simulink library "batt_packBTMSExampleLib"  (R2023a)
settings: Solver=VariableStepAuto  StartTime=0.0  StopTime=10.0  RelTol=1e-3
libraries: batt_packBTMSExampleLib_lib x12
(part 2 of 2)

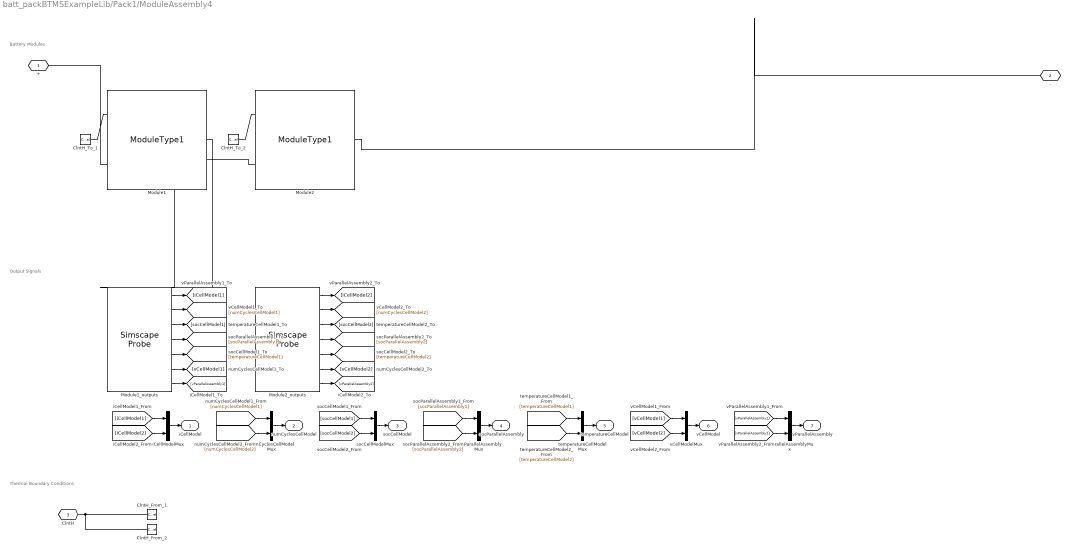
== system batt_packBTMSExampleLib/Pack1/ModuleAssembly4 ==
  note: Thermal Boundary Conditions
  note: Output Signals
  note: Battery Modules
  ClntH_From_1 : ConnectionLabel  Label=clntH_1
  ClntH_From_2 : ConnectionLabel  Label=clntH_2
  ClntH_To_1 : ConnectionLabel  Label=clntH_1
  ClntH_To_2 : ConnectionLabel  Label=clntH_2
  Module1 : batt_packBTMSExampleLib_lib/Modules/ModuleType1  SOC_vec=ModuleType1.SOC_vec  T_vec=ModuleType1.T_vec K  V0_mat=ModuleType1.V0_mat V  V_range=ModuleType1.V_range V  R0_mat=ModuleType1.R0_mat Ohm  AH=ModuleType1.AH A*hr  extrapolation_option=simscape.enum.extrapolation.nearest  thermal_mass=ModuleType1.thermal_mass J/K  CoolantThermalPathResistance=ModuleType1.CoolantThermalPathResistance K/W  P=3  S=11  iCellModel_specify=on  iCellModel_priority=None  iCellModel=ModuleAssembly4.Module1.iCellModel A  iCellModel_nominal_specify=off  iCellModel_nominal_unit=A  iCellModel_nominal_value=1  vCellModel_specify=on  vCellModel_priority=None  vCellModel=ModuleAssembly4.Module1.vCellModel V  vCellModel_nominal_specify=off  vCellModel_nominal_unit=V  vCellModel_nominal_value=1  socCellModel_specify=on  socCellModel_priority=High  socCellModel=ModuleAssembly4.Module1.socCellModel  socCellModel_nominal_specify=off  socCellModel_nominal_unit=1  socCellModel_nominal_value=1  numCyclesCellModel_specify=on  numCyclesCellModel_priority=High  numCyclesCellModel=ModuleAssembly4.Module1.numCyclesCellModel  numCyclesCellModel_nominal_specify=off  numCyclesCellModel_nominal_unit=1  numCyclesCellModel_nominal_value=1  temperatureCellModel_specify=on  temperatureCellModel_priority=High  temperatureCellModel=ModuleAssembly4.Module1.temperatureCellModel K  temperatureCellModel_nominal_specify=off  temperatureCellModel_nominal_unit=K  temperatureCellModel_nominal_value=1  vParallelAssembly_specify=on  vParallelAssembly_priority=None  vParallelAssembly=ModuleAssembly4.Module1.vParallelAssembly V  vParallelAssembly_nominal_specify=off  vParallelAssembly_nominal_unit=V  vParallelAssembly_nominal_value=1  socParallelAssembly_specify=on  socParallelAssembly_priority=None  socParallelAssembly=ModuleAssembly4.Module1.socParallelAssembly  socParallelAssembly_nominal_specify=off  socParallelAssembly_nominal_unit=1  socParallelAssembly_nominal_value=1
      settings: InternalSimscapePortConfiguration="{\"Bottom\":[{\"id\":\"n\",\"label\":\"-\",\"type\":\"foundation.electrical.electrical\"}],\"Left\":[{\"id\":\"ClntH\",\"label\":\"CH\",\"type\":\"foundation.thermal.thermal\"}],\"Right\":[],\"Top\":[{\"id\":\"p\",\"label\":\"+\",\"type\":\"foundation.electrical.electrical\"}]}"
  Module1_outputs : SimscapeProbe  BoundBlock=236  Variables={iCellModel, numCyclesCellModel, socCellModel, socParallelAssembly, temperatureCellModel, vCellModel, vParallelAssembly}
  Module2 : batt_packBTMSExampleLib_lib/Modules/ModuleType1  SOC_vec=ModuleType1.SOC_vec  T_vec=ModuleType1.T_vec K  V0_mat=ModuleType1.V0_mat V  V_range=ModuleType1.V_range V  R0_mat=ModuleType1.R0_mat Ohm  AH=ModuleType1.AH A*hr  extrapolation_option=simscape.enum.extrapolation.nearest  thermal_mass=ModuleType1.thermal_mass J/K  CoolantThermalPathResistance=ModuleType1.CoolantThermalPathResistance K/W  P=3  S=11  iCellModel_specify=on  iCellModel_priority=None  iCellModel=ModuleAssembly4.Module2.iCellModel A  iCellModel_nominal_specify=off  iCellModel_nominal_unit=A  iCellModel_nominal_value=1  vCellModel_specify=on  vCellModel_priority=None  vCellModel=ModuleAssembly4.Module2.vCellModel V  vCellModel_nominal_specify=off  vCellModel_nominal_unit=V  vCellModel_nominal_value=1  socCellModel_specify=on  socCellModel_priority=High  socCellModel=ModuleAssembly4.Module2.socCellModel  socCellModel_nominal_specify=off  socCellModel_nominal_unit=1  socCellModel_nominal_value=1  numCyclesCellModel_specify=on  numCyclesCellModel_priority=High  numCyclesCellModel=ModuleAssembly4.Module2.numCyclesCellModel  numCyclesCellModel_nominal_specify=off  numCyclesCellModel_nominal_unit=1  numCyclesCellModel_nominal_value=1  temperatureCellModel_specify=on  temperatureCellModel_priority=High  temperatureCellModel=ModuleAssembly4.Module2.temperatureCellModel K  temperatureCellModel_nominal_specify=off  temperatureCellModel_nominal_unit=K  temperatureCellModel_nominal_value=1  vParallelAssembly_specify=on  vParallelAssembly_priority=None  vParallelAssembly=ModuleAssembly4.Module2.vParallelAssembly V  vParallelAssembly_nominal_specify=off  vParallelAssembly_nominal_unit=V  vParallelAssembly_nominal_value=1  socParallelAssembly_specify=on  socParallelAssembly_priority=None  socParallelAssembly=ModuleAssembly4.Module2.socParallelAssembly  socParallelAssembly_nominal_specify=off  socParallelAssembly_nominal_unit=1  socParallelAssembly_nominal_value=1
      settings: InternalSimscapePortConfiguration="{\"Bottom\":[{\"id\":\"n\",\"label\":\"-\",\"type\":\"foundation.electrical.electrical\"}],\"Left\":[{\"id\":\"ClntH\",\"label\":\"CH\",\"type\":\"foundation.thermal.thermal\"}],\"Right\":[],\"Top\":[{\"id\":\"p\",\"label\":\"+\",\"type\":\"foundation.electrical.electrical\"}]}"
  Module2_outputs : SimscapeProbe  BoundBlock=238  Variables={iCellModel, numCyclesCellModel, socCellModel, socParallelAssembly, temperatureCellModel, vCellModel, vParallelAssembly}
  iCellModelMux : Mux  Inputs=2
  numCyclesCellModelMux : Mux  Inputs=2
  socCellModelMux : Mux  Inputs=2
  socParallelAssemblyMux : Mux  Inputs=2
  temperatureCellModelMux : Mux  Inputs=2
  vCellModelMux : Mux  Inputs=2
  vParallelAssemblyMux : Mux  Inputs=2
  + : PMIOPort  Side=Left
  - : PMIOPort  Port=2  Side=Right
  ClntH : PMIOPort  Port=3  Side=Right
  iCellModel : Outport
  numCyclesCellModel : Outport  Port=2
  socCellModel : Outport  Port=3
  socParallelAssembly : Outport  Port=4
  temperatureCellModel : Outport  Port=5
  vCellModel : Outport  Port=6
  vParallelAssembly : Outport  Port=7
  wires:
  [vParallelAssembly2] -> vParallelAssemblyMux/2
  Module2_outputs/1 -> [iCellModel2]
  [vCellModel2] -> vCellModelMux/2
  Module2_outputs/2 -> [numCyclesCellModel2]
  [temperatureCellModel2] -> temperatureCellModelMux/2
  Module2_outputs/3 -> [socCellModel2]
  [socParallelAssembly2] -> socParallelAssemblyMux/2
  Module2_outputs/4 -> [socParallelAssembly2]
  [socCellModel2] -> socCellModelMux/2
  Module2_outputs/5 -> [temperatureCellModel2]
  [numCyclesCellModel2] -> numCyclesCellModelMux/2
  Module2_outputs/6 -> [vCellModel2]
  [iCellModel2] -> iCellModelMux/2
  Module2_outputs/7 -> [vParallelAssembly2]
  [vParallelAssembly1] -> vParallelAssemblyMux/1
  vParallelAssemblyMux/1 -> vParallelAssembly/1
  Module1_outputs/1 -> [iCellModel1]
  [vCellModel1] -> vCellModelMux/1
  vCellModelMux/1 -> vCellModel/1
  Module1_outputs/2 -> [numCyclesCellModel1]
  [temperatureCellModel1] -> temperatureCellModelMux/1
  temperatureCellModelMux/1 -> temperatureCellModel/1
  Module1_outputs/3 -> [socCellModel1]
  [socParallelAssembly1] -> socParallelAssemblyMux/1
  socParallelAssemblyMux/1 -> socParallelAssembly/1
  Module1_outputs/4 -> [socParallelAssembly1]
  [socCellModel1] -> socCellModelMux/1
  socCellModelMux/1 -> socCellModel/1
  Module1_outputs/5 -> [temperatureCellModel1]
  [numCyclesCellModel1] -> numCyclesCellModelMux/1
  numCyclesCellModelMux/1 -> numCyclesCellModel/1
  Module1_outputs/6 -> [vCellModel1]
  [iCellModel1] -> iCellModelMux/1
  iCellModelMux/1 -> iCellModel/1
  Module1_outputs/7 -> [vParallelAssembly1]
  connections:
  ClntH_To_2/LConn1 -- Module2/LConn1
  ClntH_From_2/LConn1 -- ClntH_From_1/LConn1 -- ClntH/RConn1
  ClntH_To_1/LConn1 -- Module1/LConn1
  Module2/RConn1 -- -/RConn1
  Module1/LConn2 -- +/RConn1
  Module2/LConn2 -- Module1/RConn1

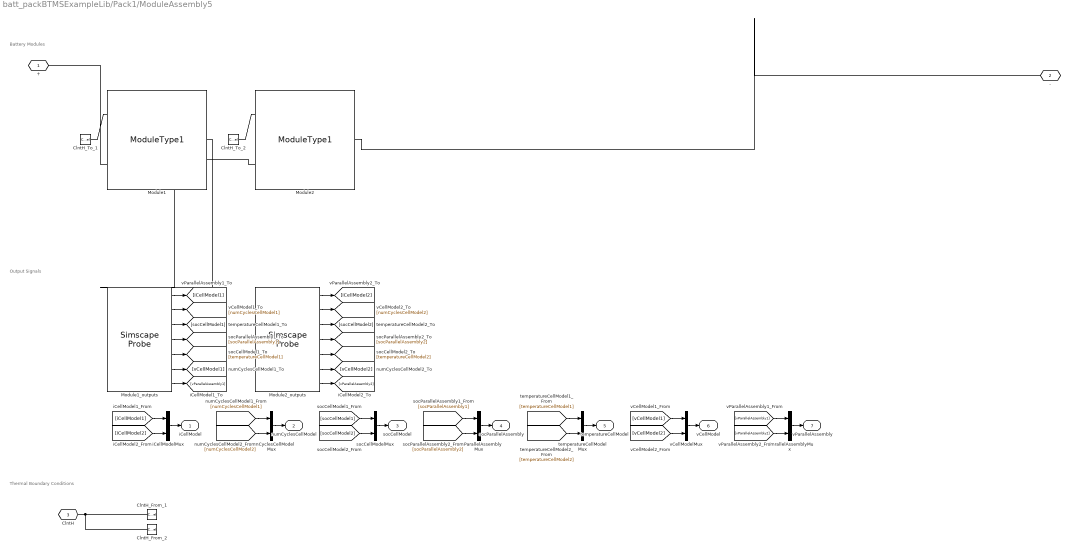
== system batt_packBTMSExampleLib/Pack1/ModuleAssembly5 ==
  note: Thermal Boundary Conditions
  note: Output Signals
  note: Battery Modules
  ClntH_From_1 : ConnectionLabel  Label=clntH_1
  ClntH_From_2 : ConnectionLabel  Label=clntH_2
  ClntH_To_1 : ConnectionLabel  Label=clntH_1
  ClntH_To_2 : ConnectionLabel  Label=clntH_2
  Module1 : batt_packBTMSExampleLib_lib/Modules/ModuleType1  SOC_vec=ModuleType1.SOC_vec  T_vec=ModuleType1.T_vec K  V0_mat=ModuleType1.V0_mat V  V_range=ModuleType1.V_range V  R0_mat=ModuleType1.R0_mat Ohm  AH=ModuleType1.AH A*hr  extrapolation_option=simscape.enum.extrapolation.nearest  thermal_mass=ModuleType1.thermal_mass J/K  CoolantThermalPathResistance=ModuleType1.CoolantThermalPathResistance K/W  P=3  S=11  iCellModel_specify=on  iCellModel_priority=None  iCellModel=ModuleAssembly5.Module1.iCellModel A  iCellModel_nominal_specify=off  iCellModel_nominal_unit=A  iCellModel_nominal_value=1  vCellModel_specify=on  vCellModel_priority=None  vCellModel=ModuleAssembly5.Module1.vCellModel V  vCellModel_nominal_specify=off  vCellModel_nominal_unit=V  vCellModel_nominal_value=1  socCellModel_specify=on  socCellModel_priority=High  socCellModel=ModuleAssembly5.Module1.socCellModel  socCellModel_nominal_specify=off  socCellModel_nominal_unit=1  socCellModel_nominal_value=1  numCyclesCellModel_specify=on  numCyclesCellModel_priority=High  numCyclesCellModel=ModuleAssembly5.Module1.numCyclesCellModel  numCyclesCellModel_nominal_specify=off  numCyclesCellModel_nominal_unit=1  numCyclesCellModel_nominal_value=1  temperatureCellModel_specify=on  temperatureCellModel_priority=High  temperatureCellModel=ModuleAssembly5.Module1.temperatureCellModel K  temperatureCellModel_nominal_specify=off  temperatureCellModel_nominal_unit=K  temperatureCellModel_nominal_value=1  vParallelAssembly_specify=on  vParallelAssembly_priority=None  vParallelAssembly=ModuleAssembly5.Module1.vParallelAssembly V  vParallelAssembly_nominal_specify=off  vParallelAssembly_nominal_unit=V  vParallelAssembly_nominal_value=1  socParallelAssembly_specify=on  socParallelAssembly_priority=None  socParallelAssembly=ModuleAssembly5.Module1.socParallelAssembly  socParallelAssembly_nominal_specify=off  socParallelAssembly_nominal_unit=1  socParallelAssembly_nominal_value=1
      settings: InternalSimscapePortConfiguration="{\"Bottom\":[{\"id\":\"n\",\"label\":\"-\",\"type\":\"foundation.electrical.electrical\"}],\"Left\":[{\"id\":\"ClntH\",\"label\":\"CH\",\"type\":\"foundation.thermal.thermal\"}],\"Right\":[],\"Top\":[{\"id\":\"p\",\"label\":\"+\",\"type\":\"foundation.electrical.electrical\"}]}"
  Module1_outputs : SimscapeProbe  BoundBlock=293  Variables={iCellModel, numCyclesCellModel, socCellModel, socParallelAssembly, temperatureCellModel, vCellModel, vParallelAssembly}
  Module2 : batt_packBTMSExampleLib_lib/Modules/ModuleType1  SOC_vec=ModuleType1.SOC_vec  T_vec=ModuleType1.T_vec K  V0_mat=ModuleType1.V0_mat V  V_range=ModuleType1.V_range V  R0_mat=ModuleType1.R0_mat Ohm  AH=ModuleType1.AH A*hr  extrapolation_option=simscape.enum.extrapolation.nearest  thermal_mass=ModuleType1.thermal_mass J/K  CoolantThermalPathResistance=ModuleType1.CoolantThermalPathResistance K/W  P=3  S=11  iCellModel_specify=on  iCellModel_priority=None  iCellModel=ModuleAssembly5.Module2.iCellModel A  iCellModel_nominal_specify=off  iCellModel_nominal_unit=A  iCellModel_nominal_value=1  vCellModel_specify=on  vCellModel_priority=None  vCellModel=ModuleAssembly5.Module2.vCellModel V  vCellModel_nominal_specify=off  vCellModel_nominal_unit=V  vCellModel_nominal_value=1  socCellModel_specify=on  socCellModel_priority=High  socCellModel=ModuleAssembly5.Module2.socCellModel  socCellModel_nominal_specify=off  socCellModel_nominal_unit=1  socCellModel_nominal_value=1  numCyclesCellModel_specify=on  numCyclesCellModel_priority=High  numCyclesCellModel=ModuleAssembly5.Module2.numCyclesCellModel  numCyclesCellModel_nominal_specify=off  numCyclesCellModel_nominal_unit=1  numCyclesCellModel_nominal_value=1  temperatureCellModel_specify=on  temperatureCellModel_priority=High  temperatureCellModel=ModuleAssembly5.Module2.temperatureCellModel K  temperatureCellModel_nominal_specify=off  temperatureCellModel_nominal_unit=K  temperatureCellModel_nominal_value=1  vParallelAssembly_specify=on  vParallelAssembly_priority=None  vParallelAssembly=ModuleAssembly5.Module2.vParallelAssembly V  vParallelAssembly_nominal_specify=off  vParallelAssembly_nominal_unit=V  vParallelAssembly_nominal_value=1  socParallelAssembly_specify=on  socParallelAssembly_priority=None  socParallelAssembly=ModuleAssembly5.Module2.socParallelAssembly  socParallelAssembly_nominal_specify=off  socParallelAssembly_nominal_unit=1  socParallelAssembly_nominal_value=1
      settings: InternalSimscapePortConfiguration="{\"Bottom\":[{\"id\":\"n\",\"label\":\"-\",\"type\":\"foundation.electrical.electrical\"}],\"Left\":[{\"id\":\"ClntH\",\"label\":\"CH\",\"type\":\"foundation.thermal.thermal\"}],\"Right\":[],\"Top\":[{\"id\":\"p\",\"label\":\"+\",\"type\":\"foundation.electrical.electrical\"}]}"
  Module2_outputs : SimscapeProbe  BoundBlock=295  Variables={iCellModel, numCyclesCellModel, socCellModel, socParallelAssembly, temperatureCellModel, vCellModel, vParallelAssembly}
  iCellModelMux : Mux  Inputs=2
  numCyclesCellModelMux : Mux  Inputs=2
  socCellModelMux : Mux  Inputs=2
  socParallelAssemblyMux : Mux  Inputs=2
  temperatureCellModelMux : Mux  Inputs=2
  vCellModelMux : Mux  Inputs=2
  vParallelAssemblyMux : Mux  Inputs=2
  + : PMIOPort  Side=Left
  - : PMIOPort  Port=2  Side=Right
  ClntH : PMIOPort  Port=3  Side=Right
  iCellModel : Outport
  numCyclesCellModel : Outport  Port=2
  socCellModel : Outport  Port=3
  socParallelAssembly : Outport  Port=4
  temperatureCellModel : Outport  Port=5
  vCellModel : Outport  Port=6
  vParallelAssembly : Outport  Port=7
  wires:
  [vParallelAssembly2] -> vParallelAssemblyMux/2
  Module2_outputs/1 -> [iCellModel2]
  [vCellModel2] -> vCellModelMux/2
  Module2_outputs/2 -> [numCyclesCellModel2]
  [temperatureCellModel2] -> temperatureCellModelMux/2
  Module2_outputs/3 -> [socCellModel2]
  [socParallelAssembly2] -> socParallelAssemblyMux/2
  Module2_outputs/4 -> [socParallelAssembly2]
  [socCellModel2] -> socCellModelMux/2
  Module2_outputs/5 -> [temperatureCellModel2]
  [numCyclesCellModel2] -> numCyclesCellModelMux/2
  Module2_outputs/6 -> [vCellModel2]
  [iCellModel2] -> iCellModelMux/2
  Module2_outputs/7 -> [vParallelAssembly2]
  [vParallelAssembly1] -> vParallelAssemblyMux/1
  vParallelAssemblyMux/1 -> vParallelAssembly/1
  Module1_outputs/1 -> [iCellModel1]
  [vCellModel1] -> vCellModelMux/1
  vCellModelMux/1 -> vCellModel/1
  Module1_outputs/2 -> [numCyclesCellModel1]
  [temperatureCellModel1] -> temperatureCellModelMux/1
  temperatureCellModelMux/1 -> temperatureCellModel/1
  Module1_outputs/3 -> [socCellModel1]
  [socParallelAssembly1] -> socParallelAssemblyMux/1
  socParallelAssemblyMux/1 -> socParallelAssembly/1
  Module1_outputs/4 -> [socParallelAssembly1]
  [socCellModel1] -> socCellModelMux/1
  socCellModelMux/1 -> socCellModel/1
  Module1_outputs/5 -> [temperatureCellModel1]
  [numCyclesCellModel1] -> numCyclesCellModelMux/1
  numCyclesCellModelMux/1 -> numCyclesCellModel/1
  Module1_outputs/6 -> [vCellModel1]
  [iCellModel1] -> iCellModelMux/1
  iCellModelMux/1 -> iCellModel/1
  Module1_outputs/7 -> [vParallelAssembly1]
  connections:
  ClntH_To_2/LConn1 -- Module2/LConn1
  ClntH_From_2/LConn1 -- ClntH_From_1/LConn1 -- ClntH/RConn1
  ClntH_To_1/LConn1 -- Module1/LConn1
  Module2/RConn1 -- -/RConn1
  Module1/LConn2 -- +/RConn1
  Module2/LConn2 -- Module1/RConn1
